simulink subsystem "drone_control"  (R2023a)
settings: Solver=VariableStepAuto  StartTime=0.0  StopTime=10.0  RelTol=1e-3
model mask{k_P=0, k_D=0}
  mask prompts: k_P "Proportional (P):"; k_D "Derivative (D):"
settings Model: Creator=User  LastModifiedBy=User

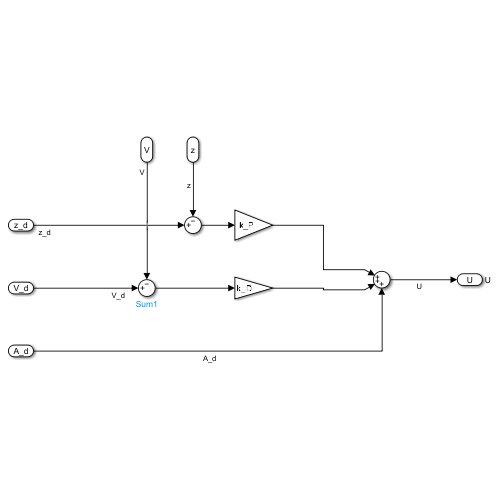
[thumbnail: Simulink's stored preview of the top-level diagram]
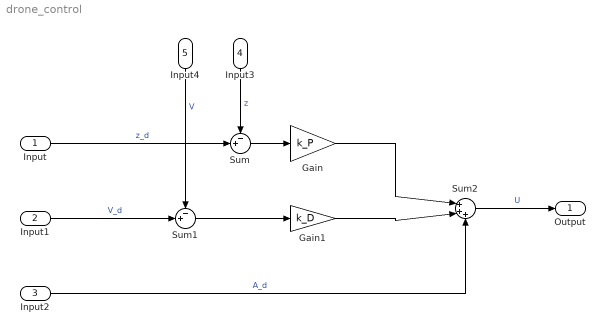
== system drone_control ==
  Input : Inport
  Input1 : Inport  Port=2
  Input2 : Inport  Port=3
  Input3 : Inport  Port=4
  Input4 : Inport  Port=5
  Gain : Gain  Gain=k_P
  Gain1 : Gain  Gain=k_D
  Sum : Sum  Inputs=-+|
  Sum1 : Sum  Inputs=-+|
  Sum2 : Sum  Inputs=|+++
  Output : Outport  SignalName=U
  wires:
  Input1/1 -> Sum1/2  "V_d"
  Input2/1 -> Sum2/3  "A_d"
  Input/1 -> Sum/2  "z_d"
  Sum/1 -> Gain/1
  Sum1/1 -> Gain1/1
  Gain/1 -> Sum2/1
  Gain1/1 -> Sum2/2
  Sum2/1 -> Output/1  "U"
  Input3/1 -> Sum/1  "z"
  Input4/1 -> Sum1/1  "V"
